simulink model "PodSimulation"  (R2020a)
settings: Solver=VariableStepAuto  StartTime=0.0  StopTime=10.0  RelTol=1e-3
settings Model: Creator=James Bates  LastModifiedBy=James Bates

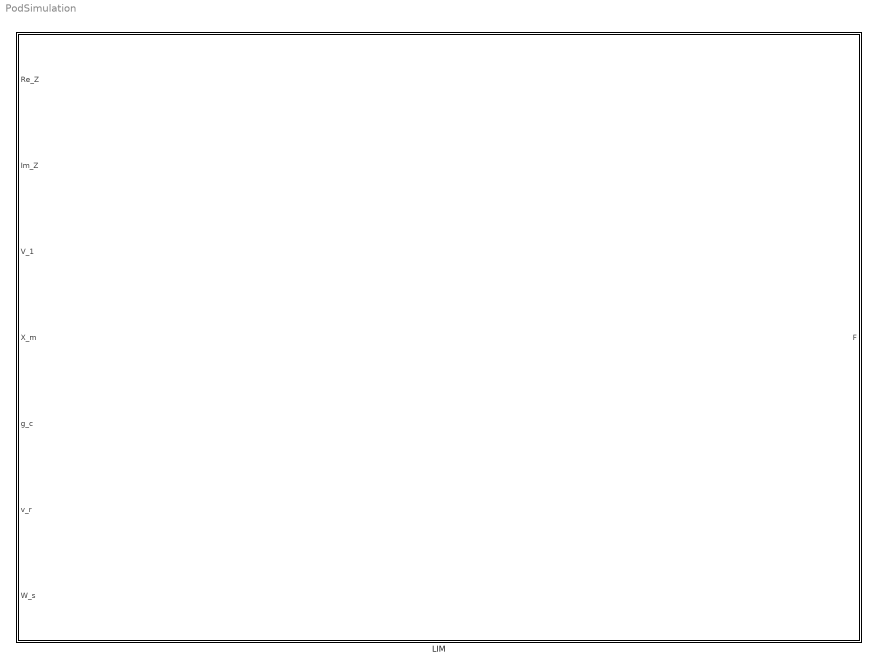
== system PodSimulation ==
  LIM : Subsystem

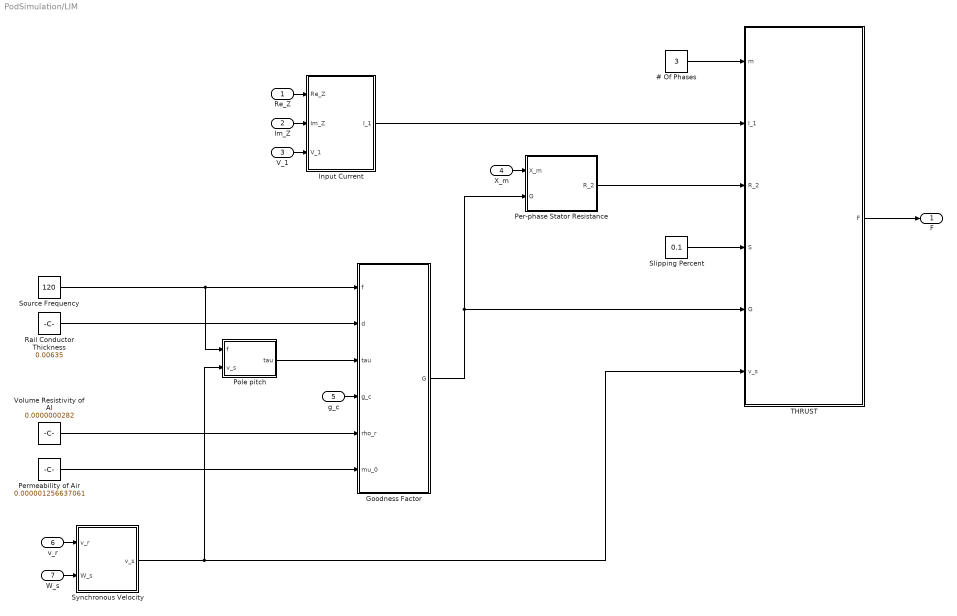
== system PodSimulation/LIM ==
  Re_Z : Inport
  Im_Z : Inport  Port=2
  V_1 : Inport  Port=3
  X_m : Inport  Port=4
  g_c : Inport  Port=5
  v_r : Inport  Port=6
  W_s : Inport  Port=7
  " Input Current" : MATLAB Function  TreatAsAtomicUnit=on
  # Of Phases : Constant  Value=3
  Goodness Factor : MATLAB Function  TreatAsAtomicUnit=on
  "Per-phase Stator Resistance " : MATLAB Function  TreatAsAtomicUnit=on
  Permeability of Air : Constant  Value=0.000001256637061
  Pole pitch : MATLAB Function  TreatAsAtomicUnit=on
  Rail Conductor Thickness : Constant  Value=0.00635
  Slipping Percent : Constant  Value=0.1
  Source Frequency : Constant  Value=120
  Synchronous Velocity : MATLAB Function  TreatAsAtomicUnit=on
  THRUST : MATLAB Function  TreatAsAtomicUnit=on
  Volume Resistivity of Al : Constant  Value=0.0000000282
  F : Outport
  wires:
  "Per-phase Stator Resistance "/1(R_2) -> THRUST/3(R_2)
  Goodness Factor/1(G) -> "Per-phase Stator Resistance "/2(G), THRUST/5(G)
  Source Frequency/1 -> Pole pitch/1(f), Goodness Factor/1(f)
  Re_Z/1 -> " Input Current"/1(Re_Z)
  # Of Phases/1 -> THRUST/1(m)
  Im_Z/1 -> " Input Current"/2(Im_Z)
  Synchronous Velocity/1(v_s) -> Pole pitch/2(v_s), THRUST/6(v_s)
  Permeability of Air/1 -> Goodness Factor/6(mu_0)
  Volume Resistivity of Al/1 -> Goodness Factor/5(rho_r)
  Slipping Percent/1 -> THRUST/4(S)
  Pole pitch/1(tau) -> Goodness Factor/3(tau)
  " Input Current"/1(I_1) -> THRUST/2(I_1)
  Rail Conductor Thickness/1 -> Goodness Factor/2(d)
  V_1/1 -> " Input Current"/3(V_1)
  W_s/1 -> Synchronous Velocity/2(W_s)
  v_r/1 -> Synchronous Velocity/1(v_r)
  X_m/1 -> "Per-phase Stator Resistance "/1(X_m)
  g_c/1 -> Goodness Factor/4(g_c)
  THRUST/1(F) -> F/1

== matlab function PodSimulation/LIM/Goodness Factor ==
  data: f input; G output; d input; tau input; g_c input; rho_r input; mu_0 input
function G = fcn(f,d,tau,g_c,rho_r,mu_0)
%f & d are Variables
% mu_0 is a Constant
G = 2*mu_0*f*tau*tau/(pi*g_c*(rho_r/d));

== matlab function PodSimulation/LIM/THRUST ==
  data: m input; F output; I_1 input; R_2 input; S input; G input; v_s input
function F = fcn(m,I_1,R_2,S,G,v_s)

F = m*(I_1*I_1)*R_2/((1/(S*S*G*G)+1)*S*v_s);

== matlab function PodSimulation/LIM/Synchronous Velocity ==
  data: v_r input; v_s output; W_s input
function v_s = fcn(v_r, W_s)
% Both inputs are variables

v_s = v_r/(1-W_s);

== matlab function PodSimulation/LIM/Per-phase Stator Resistance  ==
  data: X_m input; R_2 output; G input
function R_2 = fcn(X_m, G)

R_2 = X_m/G;

== matlab function PodSimulation/LIM/ Input Current ==
  data: Re_Z input; I_1 output; Im_Z input; V_1 input
function I_1 = fcn(Re_Z, Im_Z, V_1)
%Re_Z = Re(Z)
%Im_Z = Im(Z)

I_1 = V_1/sqrt(Re_Z*Re_Z+Im_Z*Im_Z);

== matlab function PodSimulation/LIM/Pole pitch ==
  data: f input; tau output; v_s input
function tau = fcn(f, v_s)

tau = v_s/(2*f);
